simulink model "VCU_Software_Harness1"  (R2025b)
settings: Solver=FixedStepDiscrete  StartTime=0  StopTime=2474  FixedStep=0.01  RelTol=2e-1  AbsTol=1e-1
undefined symbols (not defined in the file): Drv_Mode, m
libraries: SignalEditorBlockLib x1
settings Model: DataDictionary=VirtualVehicleTemplate.sldd  Creator=smuckati  LastModifiedBy=jghidell
settings SolverCC: AutoScaleAbsTol=off  SolverJacobianMethodControl=FullPerturbation  ZeroCrossAlgorithm=Adaptive  AlgebraicLoopSolver=TrustRegion  AutoInsertRateTranBlk=on  InsertRTBMode=Never (minimum delay)  DecoupledContinuousIntegration=on  MinimalZcImpactIntegration=on  MaxZcPerStep=1.0
settings OptimizationCC: DefaultParameterBehavior=Inlined  UseDivisionForNetSlopeComputation=on  GainParamInheritBuiltInType=on  UseFloatMulNetSlope=on  UseSpecifiedMinMax=on  InlineInvariantSignals=on  BitwiseOrLogicalOp=Bitwise operator  PassReuseOutputArgsAs=Individual arguments  ZeroExternalMemoryAtStartup=off  ZeroInternalMemoryAtStartup=off  NoFixptDivByZeroProtection=on  EfficientFloat2IntCast=on  LifeSpan=1  OptimizeBlockOrder=speed  DifferentSizesBufferReuse=on  EfficientTunableParamExpr=on
settings DebuggingCC: SignalInfNanChecking=error  ArtificialAlgebraicLoopMsg=none  MaskedZcDiagnostic=none  IgnoredZcDiagnostic=none  ParameterTunabilityLossMsg=error  UnconnectedInputMsg=warning  UnconnectedOutputMsg=warning  UnconnectedLineMsg=warning  PregeneratedLibrarySubsystemCodeDiagnostic=none  SubsystemReferenceDiagnosticForUnitTest=warning  ArithmeticOperatorsInVariantConditions=warning
settings HardwareCC: ProdBitPerPointer=32.0  ProdBitPerSizeT=32.0  ProdBitPerPtrDiffT=32.0  ProdLargestAtomicFloat=None  ProdWordSize=32.0  ProdHWDeviceType=Custom Processor->Custom Processor
settings ModelReferenceCC: UpdateModelReferenceTargets=IfOutOfDate  EnableRefExpFcnMdlSchedulingChecks=on  ModelReferenceMinAlgLoopOccurrences=on  PropagateSignalLabelsOutOfModel=off
settings SFSimCC: SimUseLocalCustomCode=off  SimGenImportedTypeDefs=on  MATLABDynamicMemAlloc=off  SimTargetLang=C++  SimDLTargetLibrary=mkl-dnn
settings RTWCC: SystemTargetFile=autosar_adaptive.tlc  GenCodeOnly=on  PackageGeneratedCodeAndArtifacts=on  TemplateMakefile=ert_default_tmf  GenerateReport=on  RTWUseLocalCustomCode=off  Toolchain=AUTOSAR Adaptive | CMake  BuildConfiguration=Release  IncludeHyperlinkInReport=on  DataTypeReplacement=CDataTypesFixedWidth  TargetLang=C++  GenerateTraceInfo=on  GenerateTraceReport=on  GenerateTraceReportSl=on  GenerateTraceReportSf=on  GenerateTraceReportEml=on  GenerateCodeMetricsReport=on  GenerateCodeReplacementReport=on  GPUComputeCapability=3.5  DLArmComputeVersion=19.05  Description=AUTOSAR Adaptive
settings CodeAppCC: ForceParamTrailComments=on  IgnoreCustomStorageClasses=off  MaxIdLength=63.0  OperatorAnnotations=on  SimulinkDataObjDesc=on  SFDataObjDesc=on  CustomSymbolStrGlobalVar=rt$N$M  CustomSymbolStrType=$N$M  CustomSymbolStrFcn=$N$M$F  CustomSymbolStrMacro=$N$M  InsertBlockDesc=on
settings AUTOSARAdaptiveTargetCC: AutosarSchemaVersion=R20-11  AutosarMaxShortNameLength=128.0  AdaptiveAutosarXCPServerTransportLayer=None  AdaptiveAutosarXCPServerTCPIPAddress=127.0.0.1  AdaptiveAutosarXCPServerPort=17725  AdaptiveAutosarXCPServerVerbosity=off  AdaptiveAutosarUseCustomXCPServer=off  DSAsUniqueAccess=off  ExtMode=off  ExtModeTransport=0.0  ExtModeStaticAlloc=off  ExtModeAutomaticAllocSize=on  ExtModeMaxTrigDuration=10.0  ExtModeStaticAllocSize=1000000.0  ExtModeTesting=off  ExtModeMexFile=ext_comm  ExtModeIntrfLevel=Level1  InlinedParameterPlacement=NonHierarchical  TargetOS=BareBoardExample  MultiInstanceErrorCode=Error  RootIOFormat=Structure reference  SubcomponentRootIOFormat=Auto  RTWCAPISignals=off  RTWCAPIParams=off  RTWCAPIStates=off  RTWCAPIRootIO=off  ERTSrcFileBannerTemplate=ert_code_template.cgt  ERTHdrFileBannerTemplate=ert_code_template.cgt  ERTDataSrcFileTemplate=ert_code_template.cgt  ERTDataHdrFileTemplate=ert_code_template.cgt  ERTCustomFileTemplate=example_file_process.tlc  EnableDataOwnership=off  SignalDisplayLevel=10.0  ParamTuneLevel=10.0  GlobalDataDefinition=Auto  DataDefinitionFile=global.c  GlobalDataReference=Auto  ERTFilePackagingFormat=CompactWithDataFile  RateTransitionBlockCode=Inline  DataReferenceFile=global.h  PreserveExpressionOrder=off  PreserveIfCondition=off  ConvertIfToSwitch=on  PreserveExternInFcnDecls=on  PreserveStaticInFcnDecls=on  SuppressUnreachableDefaultCases=on  EnableSignedLeftShifts=on  EnableSignedRightShifts=on  ImplementImageWithCVMat=off  IndentStyle=K&R  IndentSize=2  NewlineStyle=Default  MaxLineWidth=80.0  EnableUserReplacementTypes=off  MaxIdInt64=INT64_MAX  MinIdInt64=INT64_MIN  MaxIdUint64=UINT64_MAX  MaxIdInt32=INT32_MAX  MinIdInt32=INT32_MIN  MaxIdUint32=UINT32_MAX  MaxIdInt16=INT16_MAX  MinIdInt16=INT16_MIN  MaxIdUint16=UINT16_MAX  MaxIdInt8=INT8_MAX  MinIdInt8=INT8_MIN  MaxIdUint8=UINT8_MAX  BooleanTrueId=true  BooleanFalseId=false  MemSecPackage=--- None ---  MemSecDataConstants=Default  MemSecDataIO=Default  MemSecDataInternal=Default  MemSecDataParameters=Default  MemSecFuncInitTerm=Default  MemSecFuncExecute=Default  MemSecFuncSharedUtil=Default  GroupConstants=Default  GroupRootInputs=Default  GroupRootOutputs=Default  GroupInternal=Default  GroupParameters=Default  GroupDataTransfer=Default  GroupSharedLocalDataStores=Default  GroupInstanceSpecificParameters=Default  GroupModelData=Default  ArrayContainerType=std::array  DynamicArrayContainerType=coder::array  TargetFcnLib=ansi_tfl_table_tmw.mat  GenFloatMathFcnCalls=NOT IN USE  TargetLangStandard=C++11 (ISO)  CodeReplacementLibrary=C++ Standard Library Mutex  UtilityFuncGeneration=Auto  MultiwordTypeDef=System defined  MultiwordLength=2048.0  DynamicStringBufferSize=256.0  GenerateFullHeader=on  InferredTypesCompatibility=off  GenerateSampleERTMain=off  GenerateTestInterfaces=off  ModelReferenceCompliant=on  ParMdlRefBuildCompliant=on  CompOptLevelCompliant=on  ConcurrentExecutionCompliant=on  IncludeMdlTerminateFcn=on  CombineOutputUpdateFcns=on  CombineSignalStateStructs=on  GroupInternalDataByFunction=off  SuppressErrorStatus=on  IncludeFileDelimiter=Auto  ERTCustomFileBanners=off  SupportAbsoluteTime=off  LogVarNameModifier=rt_  MatFileLogging=off  PreserveMATLABNamespacesInGeneratedCode=on  CodeInterfacePackaging=C++ class  SubcomponentCodeInterfacePackaging=C++ class  PurelyIntegerCode=off  SupportNonFinite=off  SupportComplex=off  SupportContinuousTime=off  SupportNonInlinedSFcns=off  RemoveDisableFunc=off  RemoveResetFunc=on  SupportVariableSizeSignals=off  ParenthesesLevel=Nominal  CastingMode=Nominal  MATLABClassNameForMDSCustomization=Simulink.SoftwareTarget.TargetSpecificTriggerConfigurationBase  ModelStepFunctionPrototypeControlCompliant=off  CPPClassGenCompliant=on  AutosarCompliant=on  MDXCompliant=off  GRTInterface=off  GenerateAllocFcn=off  UseToolchainInfoCompliant=on  GenerateSharedConstants=on  CoderGroups=[]  AccessMethods=[]  LookupTableObjectStructAxisOrder=2,1,3,4,...  LUTObjectStructOrderExplicitValues=Size,Breakpoints,Table  LUTObjectStructOrderEvenSpacing=Size,Table,Breakpoints  ArrayLayout=Column-major  UnsupportedSFcnMsg=error  ERTHeaderFileRootName=$R$E  ERTSourceFileRootName=$R$E  ERTDataFileRootName=$R_data  InstructionSetFMA=off  OptimizeReductions=off  LogToMDFFile=off

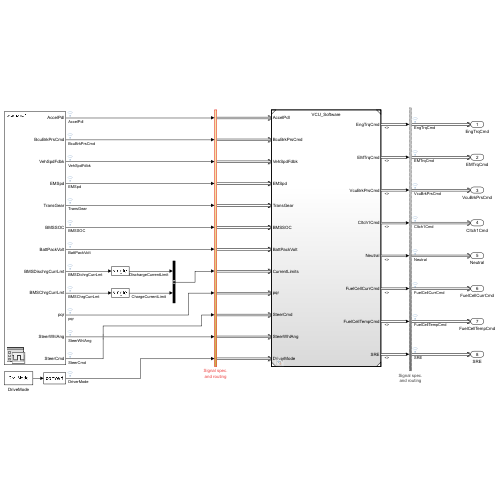
[thumbnail: Simulink's stored preview of the top-level diagram]
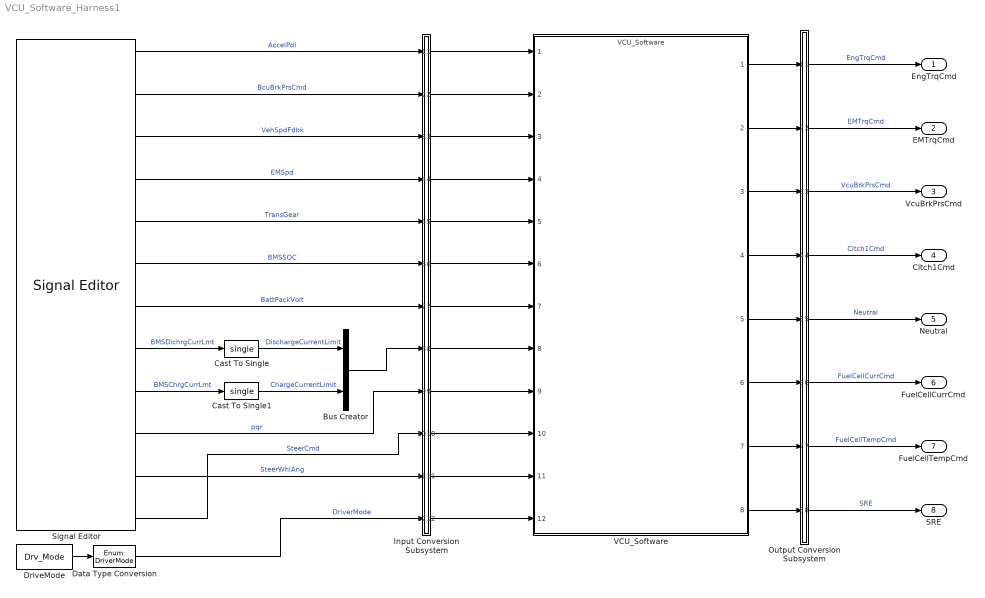
== system VCU_Software_Harness1 ==
  Bus Creator : BusCreator  Inputs=2
  Cast To Single : DataTypeConversion  OutDataTypeStr=single  SaturateOnIntegerOverflow=off  RndMeth=Floor
  Cast To Single1 : DataTypeConversion  OutDataTypeStr=single  SaturateOnIntegerOverflow=off  RndMeth=Floor
  Data Type Conversion : DataTypeConversion  OutDataTypeStr=Enum: DriverMode  SaturateOnIntegerOverflow=off  RndMeth=Floor
  DriveMode : Constant  Value=Drv_Mode  OutDataTypeStr=int8
  Input Conversion Subsystem : Subsystem  Tag=__SLT_ICS__  Description=|
      | Signal spec.
      | and routing
      settings: AttributesFormatString=%<Description>
  Output Conversion Subsystem : Subsystem  Tag=__SLT_OCS__  Description=|
      | Signal spec.
      | and routing
      settings: AttributesFormatString=%<Description>
  Signal Editor : SignalEditorBlockLib/Signal Editor  FileName=VCU_Inpts.mat  ActiveScenario=Scenario1  ActiveSignal=SteerCmd  IsBus=off  OutputBusObjectStr=Bus: BusObject  SampleTime=0.01  Interpolate=off  ZeroCross=off  OutputAfterFinalValue=Setting to zero  Unit=inherit  PreserveSignalName=on  ApplySigPropsToAllScenarios=on  ApplySigPropsToAllSignals=off  SignalPropertySource=Dialog parameters
  VCU_Software : ModelReference  InputPortMessageModes=m,m,m,m,m,m,m,m,m,m,m,m  OutputPortMessageModes=m,m,m,m,m,m,m,m  ModelNameDialog=VCU_Software  SimulationMode=Normal  ModelReferenceVersion=6.0
  EngTrqCmd : Outport  InputPortMessageModes=m
  EMTrqCmd : Outport  InputPortMessageModes=m  Port=2
  VcuBrkPrsCmd : Outport  InputPortMessageModes=m  Port=3
  Cltch1Cmd : Outport  InputPortMessageModes=m  Port=4
  Neutral : Outport  InputPortMessageModes=m  Port=5
  FuelCellCurrCmd : Outport  InputPortMessageModes=m  Port=6
  FuelCellTempCmd : Outport  InputPortMessageModes=m  Port=7
  SRE : Outport  InputPortMessageModes=m  Port=8
  wires:
  Output Conversion Subsystem/1(Outport_1) -> EngTrqCmd/1  "EngTrqCmd"
  Output Conversion Subsystem/2(Outport_2) -> EMTrqCmd/1  "EMTrqCmd"
  Output Conversion Subsystem/3(Outport_3) -> VcuBrkPrsCmd/1  "VcuBrkPrsCmd"
  Output Conversion Subsystem/4(Outport_4) -> Cltch1Cmd/1  "Cltch1Cmd"
  Output Conversion Subsystem/5(Outport_5) -> Neutral/1  "Neutral"
  Output Conversion Subsystem/6(Outport_6) -> FuelCellCurrCmd/1  "FuelCellCurrCmd"
  Output Conversion Subsystem/7(Outport_7) -> FuelCellTempCmd/1  "FuelCellTempCmd"
  Output Conversion Subsystem/8(Outport_8) -> SRE/1  "SRE"
  Signal Editor/10 -> Input Conversion Subsystem/9(Inport_9)  "pqr"
  Signal Editor/12 -> Input Conversion Subsystem/10(Inport_10)  "SteerCmd"
  Signal Editor/1 -> Input Conversion Subsystem/1(Inport_1)  "AccelPdl"
  Signal Editor/2 -> Input Conversion Subsystem/2(Inport_2)  "BcuBrkPrsCmd"
  Signal Editor/3 -> Input Conversion Subsystem/3(Inport_3)  "VehSpdFdbk"
  Signal Editor/4 -> Input Conversion Subsystem/4(Inport_4)  "EMSpd"
  Signal Editor/5 -> Input Conversion Subsystem/5(Inport_5)  "TransGear"
  Signal Editor/6 -> Input Conversion Subsystem/6(Inport_6)  "BMSSOC"
  Signal Editor/7 -> Input Conversion Subsystem/7(Inport_7)  "BattPackVolt"
  Signal Editor/8 -> Cast To Single/1  "BMSDichrgCurrLmt"
  Signal Editor/9 -> Cast To Single1/1  "BMSChrgCurrLmt"
  DriveMode/1 -> Data Type Conversion/1
  Data Type Conversion/1 -> Input Conversion Subsystem/12(Inport_12)  "DriverMode"
  Signal Editor/11 -> Input Conversion Subsystem/11(Inport_11)  "SteerWhlAng"
  VCU_Software/1 -> Output Conversion Subsystem/1(Inport_1)
  VCU_Software/2 -> Output Conversion Subsystem/2(Inport_2)
  VCU_Software/3 -> Output Conversion Subsystem/3(Inport_3)
  VCU_Software/4 -> Output Conversion Subsystem/4(Inport_4)
  VCU_Software/5 -> Output Conversion Subsystem/5(Inport_5)
  VCU_Software/6 -> Output Conversion Subsystem/6(Inport_6)
  VCU_Software/7 -> Output Conversion Subsystem/7(Inport_7)
  VCU_Software/8 -> Output Conversion Subsystem/8(Inport_8)
  Input Conversion Subsystem/1(Outport_1) -> VCU_Software/1
  Input Conversion Subsystem/2(Outport_2) -> VCU_Software/2
  Input Conversion Subsystem/3(Outport_3) -> VCU_Software/3
  Input Conversion Subsystem/4(Outport_4) -> VCU_Software/4
  Input Conversion Subsystem/5(Outport_5) -> VCU_Software/5
  Input Conversion Subsystem/6(Outport_6) -> VCU_Software/6
  Input Conversion Subsystem/7(Outport_7) -> VCU_Software/7
  Input Conversion Subsystem/8(Outport_8) -> VCU_Software/8
  Input Conversion Subsystem/9(Outport_9) -> VCU_Software/9
  Input Conversion Subsystem/10(Outport_10) -> VCU_Software/10
  Input Conversion Subsystem/11(Outport_11) -> VCU_Software/11
  Input Conversion Subsystem/12(Outport_12) -> VCU_Software/12
  Bus Creator/1 -> Input Conversion Subsystem/8(Inport_8)
  Cast To Single/1 -> Bus Creator/1  "DischargeCurrentLimit"
  Cast To Single1/1 -> Bus Creator/2  "ChargeCurrentLimit"

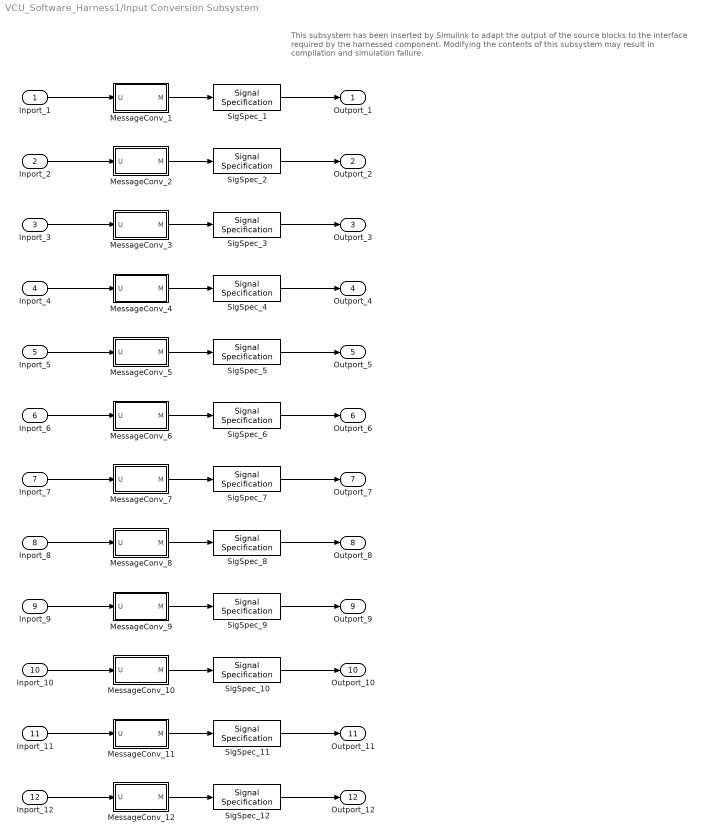
== system VCU_Software_Harness1/Input Conversion Subsystem ==
  note: This subsystem has been inserted by Simulink to adapt the output of the source blocks to the interface required by the harnessed component.
      |  Modifying the contents of this subsystem may result in compilation and simulation failure.
  Inport_1 : Inport
  Inport_2 : Inport  Port=2
  Inport_3 : Inport  Port=3
  Inport_4 : Inport  Port=4
  Inport_5 : Inport  Port=5
  Inport_6 : Inport  Port=6
  Inport_7 : Inport  Port=7
  Inport_8 : Inport  Port=8
  Inport_9 : Inport  Port=9
  Inport_10 : Inport  Port=10
  Inport_11 : Inport  Port=11
  Inport_12 : Inport  Port=12
  MessageConv_1 : Stateflow chart  TreatAsAtomicUnit=on
  MessageConv_10 : Stateflow chart  TreatAsAtomicUnit=on
  MessageConv_11 : Stateflow chart  TreatAsAtomicUnit=on
  MessageConv_12 : Stateflow chart  TreatAsAtomicUnit=on
  MessageConv_2 : Stateflow chart  TreatAsAtomicUnit=on
  MessageConv_3 : Stateflow chart  TreatAsAtomicUnit=on
  MessageConv_4 : Stateflow chart  TreatAsAtomicUnit=on
  MessageConv_5 : Stateflow chart  TreatAsAtomicUnit=on
  MessageConv_6 : Stateflow chart  TreatAsAtomicUnit=on
  MessageConv_7 : Stateflow chart  TreatAsAtomicUnit=on
  MessageConv_8 : Stateflow chart  TreatAsAtomicUnit=on
  MessageConv_9 : Stateflow chart  TreatAsAtomicUnit=on
  SigSpec_{1,3,5..7,10} (6 alike) : SignalSpecification  OutDataTypeStr=double  Dimensions=[1]  SampleTime=0.01
  SigSpec_11 : SignalSpecification  OutDataTypeStr=double  Dimensions=[4]  SampleTime=0.01
  SigSpec_12 : SignalSpecification  OutDataTypeStr=Enum: DriverMode  Dimensions=[1]  SampleTime=0.01
  SigSpec_2 : SignalSpecification  OutDataTypeStr=double  Dimensions=[4]  SampleTime=0.01
  SigSpec_4 : SignalSpecification  OutDataTypeStr=double  Dimensions=[2]  SampleTime=0.01
  SigSpec_8 : SignalSpecification  OutDataTypeStr=Bus: BattCurLims  Dimensions=[1]  BusOutputAsStruct=on
  SigSpec_9 : SignalSpecification  OutDataTypeStr=double  Dimensions=[3]  SampleTime=0.01
  Outport_1 : Outport
  Outport_2 : Outport  Port=2
  Outport_3 : Outport  Port=3
  Outport_4 : Outport  Port=4
  Outport_5 : Outport  Port=5
  Outport_6 : Outport  Port=6
  Outport_7 : Outport  Port=7
  Outport_8 : Outport  Port=8
  Outport_9 : Outport  Port=9
  Outport_10 : Outport  Port=10
  Outport_11 : Outport  Port=11
  Outport_12 : Outport  Port=12
  wires:
  SigSpec_1/1 -> Outport_1/1
  MessageConv_1/1(M) -> SigSpec_1/1
  Inport_1/1 -> MessageConv_1/1(U)
  SigSpec_2/1 -> Outport_2/1
  MessageConv_2/1(M) -> SigSpec_2/1
  Inport_2/1 -> MessageConv_2/1(U)
  SigSpec_3/1 -> Outport_3/1
  MessageConv_3/1(M) -> SigSpec_3/1
  Inport_3/1 -> MessageConv_3/1(U)
  SigSpec_4/1 -> Outport_4/1
  MessageConv_4/1(M) -> SigSpec_4/1
  Inport_4/1 -> MessageConv_4/1(U)
  SigSpec_5/1 -> Outport_5/1
  MessageConv_5/1(M) -> SigSpec_5/1
  Inport_5/1 -> MessageConv_5/1(U)
  SigSpec_6/1 -> Outport_6/1
  MessageConv_6/1(M) -> SigSpec_6/1
  Inport_6/1 -> MessageConv_6/1(U)
  SigSpec_7/1 -> Outport_7/1
  MessageConv_7/1(M) -> SigSpec_7/1
  Inport_7/1 -> MessageConv_7/1(U)
  SigSpec_8/1 -> Outport_8/1
  MessageConv_8/1(M) -> SigSpec_8/1
  Inport_8/1 -> MessageConv_8/1(U)
  SigSpec_9/1 -> Outport_9/1
  MessageConv_9/1(M) -> SigSpec_9/1
  Inport_9/1 -> MessageConv_9/1(U)
  SigSpec_10/1 -> Outport_10/1
  MessageConv_10/1(M) -> SigSpec_10/1
  Inport_10/1 -> MessageConv_10/1(U)
  SigSpec_11/1 -> Outport_11/1
  MessageConv_11/1(M) -> SigSpec_11/1
  Inport_11/1 -> MessageConv_11/1(U)
  SigSpec_12/1 -> Outport_12/1
  MessageConv_12/1(M) -> SigSpec_12/1
  Inport_12/1 -> MessageConv_12/1(U)

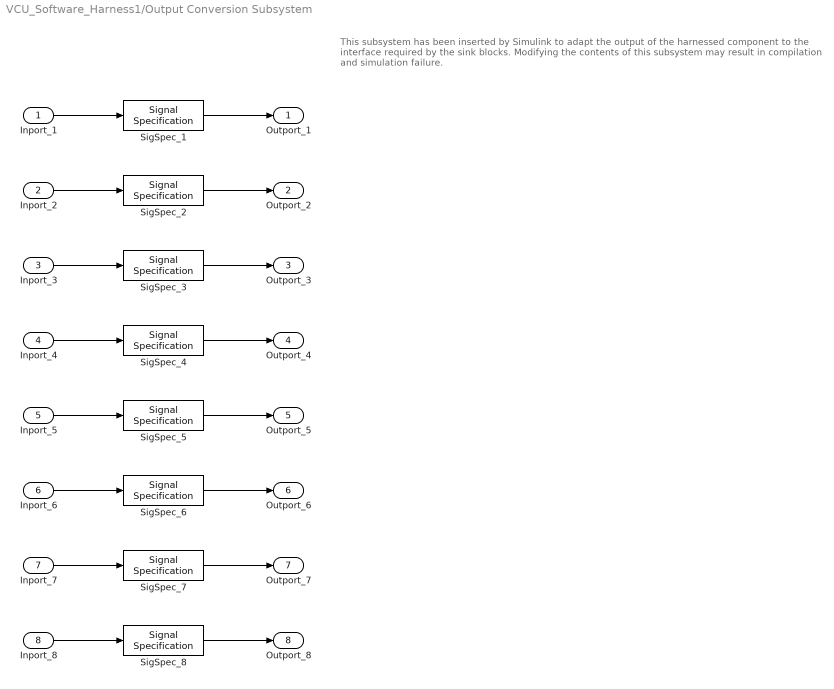
== system VCU_Software_Harness1/Output Conversion Subsystem ==
  note: This subsystem has been inserted by Simulink to adapt the output of the harnessed component to the interface required by the sink blocks.
      |  Modifying the contents of this subsystem may result in compilation and simulation failure.
  Inport_1 : Inport
  Inport_2 : Inport  Port=2
  Inport_3 : Inport  Port=3
  Inport_4 : Inport  Port=4
  Inport_5 : Inport  Port=5
  Inport_6 : Inport  Port=6
  Inport_7 : Inport  Port=7
  Inport_8 : Inport  Port=8
  SigSpec_{1,4..7} (5 alike) : SignalSpecification  OutDataTypeStr=double  Dimensions=[1]  SampleTime=0.01
  SigSpec_2 : SignalSpecification  OutDataTypeStr=double  Dimensions=[2]  SampleTime=0.01
  SigSpec_3 : SignalSpecification  OutDataTypeStr=double  Dimensions=[4]  SampleTime=0.01
  SigSpec_8 : SignalSpecification  OutDataTypeStr=Enum: SRE  Dimensions=[1]  SampleTime=0.01
  Outport_1 : Outport
  Outport_2 : Outport  Port=2
  Outport_3 : Outport  Port=3
  Outport_4 : Outport  Port=4
  Outport_5 : Outport  Port=5
  Outport_6 : Outport  Port=6
  Outport_7 : Outport  Port=7
  Outport_8 : Outport  Port=8
  wires:
  Inport_1/1 -> SigSpec_1/1
  SigSpec_1/1 -> Outport_1/1
  Inport_2/1 -> SigSpec_2/1
  SigSpec_2/1 -> Outport_2/1
  Inport_3/1 -> SigSpec_3/1
  SigSpec_3/1 -> Outport_3/1
  Inport_4/1 -> SigSpec_4/1
  SigSpec_4/1 -> Outport_4/1
  Inport_5/1 -> SigSpec_5/1
  SigSpec_5/1 -> Outport_5/1
  Inport_6/1 -> SigSpec_6/1
  SigSpec_6/1 -> Outport_6/1
  Inport_7/1 -> SigSpec_7/1
  SigSpec_7/1 -> Outport_7/1
  Inport_8/1 -> SigSpec_8/1
  SigSpec_8/1 -> Outport_8/1

== stateflow chart VCU_Software_Harness1/Input Conversion Subsystem/MessageConv_1 ==
  (default) -> (junction 10) : {M.data = U; send(M);}
  data: M output; U input

== stateflow chart VCU_Software_Harness1/Input Conversion Subsystem/MessageConv_2 ==
  (default) -> (junction 10) : {M.data = U; send(M);}
  data: M output; U input

== stateflow chart VCU_Software_Harness1/Input Conversion Subsystem/MessageConv_3 ==
  (default) -> (junction 10) : {M.data = U; send(M);}
  data: M output; U input

== stateflow chart VCU_Software_Harness1/Input Conversion Subsystem/MessageConv_4 ==
  (default) -> (junction 10) : {M.data = U; send(M);}
  data: M output; U input

== stateflow chart VCU_Software_Harness1/Input Conversion Subsystem/MessageConv_5 ==
  (default) -> (junction 10) : {M.data = U; send(M);}
  data: M output; U input

== stateflow chart VCU_Software_Harness1/Input Conversion Subsystem/MessageConv_6 ==
  (default) -> (junction 10) : {M.data = U; send(M);}
  data: M output; U input

== stateflow chart VCU_Software_Harness1/Input Conversion Subsystem/MessageConv_7 ==
  (default) -> (junction 10) : {M.data = U; send(M);}
  data: M output; U input

== stateflow chart VCU_Software_Harness1/Input Conversion Subsystem/MessageConv_8 ==
  (default) -> (junction 10) : {M.data = U; send(M);}
  data: M output Bus: BattCurLims; U input Bus: BattCurLims

== stateflow chart VCU_Software_Harness1/Input Conversion Subsystem/MessageConv_9 ==
  (default) -> (junction 10) : {M.data = U; send(M);}
  data: M output; U input

== stateflow chart VCU_Software_Harness1/Input Conversion Subsystem/MessageConv_10 ==
  (default) -> (junction 10) : {M.data = U; send(M);}
  data: M output; U input

== stateflow chart VCU_Software_Harness1/Input Conversion Subsystem/MessageConv_11 ==
  (default) -> (junction 10) : {M.data = U; send(M);}
  data: M output; U input

== stateflow chart VCU_Software_Harness1/Input Conversion Subsystem/MessageConv_12 ==
  (default) -> (junction 10) : {M.data = U; send(M);}
  data: M output; U input
